simulink model "Three_phase_mf44"  (R2023b)
settings: Solver=ode45  StartTime=0.0  StopTime=0.1  RelTol=1e-3
libraries: spsDiodeLib x6, spsIdealSwitchLib x6, spsTriangleGeneratorLib x3, spsCurrentMeasurementLib x1, spsDCVoltageSourceLib x1, spsThreePhaseSeriesRLCBranchLib x1, spsVoltageMeasurementLib x1, spspowerguiLib x1
settings Model: Creator=LX  LastModifiedBy=Ngsanchong
settings DataIOCC: ReturnWorkspaceOutputs=off

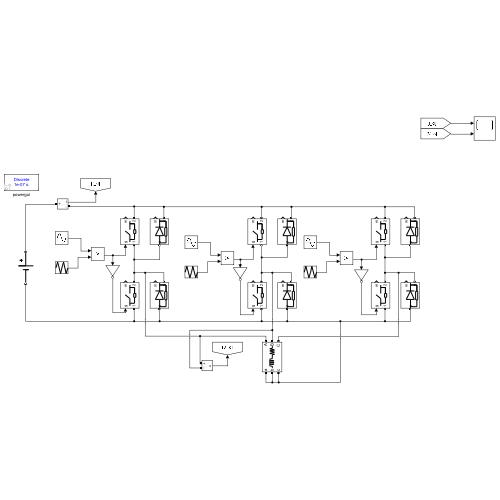
[thumbnail: Simulink's stored preview of the top-level diagram]
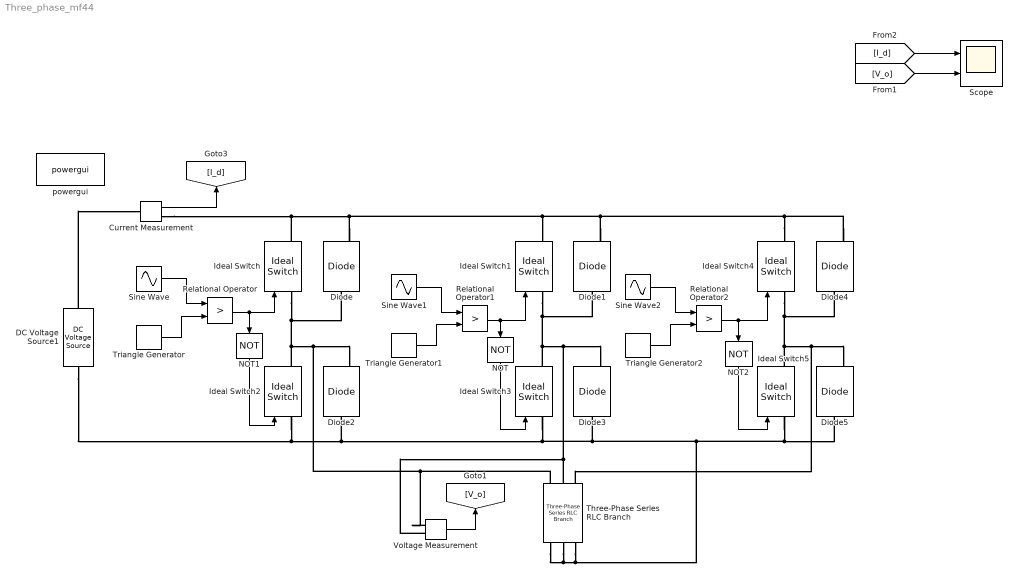
== system Three_phase_mf44 ==
  Current Measurement : spsCurrentMeasurementLib/Current Measurement  PhasorSimulation=off  OutputType=Complex  PSBequivalent=0
  DC Voltage Source1 : spsDCVoltageSourceLib/DC Voltage Source  Amplitude=540  Measurements=None
  Diode{,1..5} (6 alike) : spsDiodeLib/Diode  Ron=0.001  Lon=0  Vf=0.8  IC=0  UseSnubber=0  Rs=500  Cs=250e-9  Measurements=on
  Ideal Switch{,1..5} (6 alike) : spsIdealSwitchLib/Ideal Switch  Ron=1e-9  Lon=0  IC=0  Rs=1e5  Cs=inf  Measurements=on
  NOT : Logic  Operator=NOT  IconShape=distinctive  AllPortsSameDT=off  OutDataTypeStr=boolean
  NOT1 : Logic  Operator=NOT  IconShape=distinctive  AllPortsSameDT=off  OutDataTypeStr=boolean
  NOT2 : Logic  Operator=NOT  IconShape=distinctive  AllPortsSameDT=off  OutDataTypeStr=boolean
  Relational Operator : RelationalOperator  Operator=>  OutDataTypeStr=boolean  RndMeth=Simplest  InputSameDT=off
  Relational Operator1 : RelationalOperator  Operator=>  OutDataTypeStr=boolean  RndMeth=Simplest  InputSameDT=off
  Relational Operator2 : RelationalOperator  Operator=>  OutDataTypeStr=boolean  RndMeth=Simplest  InputSameDT=off
  Scope : Scope  NumInputPorts=2
  Sine Wave : Sin  Amplitude=1.2  Frequency=2*pi*50  SampleTime=0
  Sine Wave1 : Sin  Amplitude=1.2  Frequency=2*pi*50  Phase=-2*pi/3  SampleTime=0
  Sine Wave2 : Sin  Amplitude=1.2  Frequency=2*pi*50  Phase=2*pi/3  SampleTime=0
  Three-Phase Series RLC Branch : spsThreePhaseSeriesRLCBranchLib/Three-Phase Series RLC Branch  LConnTagsString=A|B|C  RConnTagsString=A|B|C  BranchType=RL  Resistance=5  Inductance=5e-3  Capacitance=1e-6  Measurements=None
  Triangle Generator : spsTriangleGeneratorLib/Triangle Generator  Freq=2200  Phase=90  Ts=0
  Triangle Generator1 : spsTriangleGeneratorLib/Triangle Generator  Freq=2200  Phase=90  Ts=0
  Triangle Generator2 : spsTriangleGeneratorLib/Triangle Generator  Freq=2200  Phase=90  Ts=0
  Voltage Measurement : spsVoltageMeasurementLib/Voltage Measurement  PhasorSimulation=off  OutputType=Complex  PSBequivalent=0
  powergui : spspowerguiLib/powergui  Priority=1  SimulationMode=Discrete  SampleTime=1e-7  frequency=60  Iterations=50  frequencyindice=0  Pbase=100e6  ErrMax=1e-4  UnitsV=kV  UnitsW=MW  buscounter=0  FunctionMessages=off  echomessages=off  EnableUseOfTLC=off  CurrentSourceSwitches=off  DisableSnubberDevices=off  DisableRonSwitches=off  DisableVfSwitches=off  DisplayEquations=off  AutomaticDiscreteSolvers=off  SolverType=Tustin/Backward Euler (TBE)  Interpol=off  ExternalGateDelay=off  methode=off  Ts=100  x0status=blocks  SPID=on  SwTol=0  HookPort=off  NonlinearTolerance=1e-4  nMaxIteration=100  ContinueOnMaxIteration=off  RestoreLinks=warning  ResistiveCurrentMeasurement=off  Frange=[0:2:500]  Ylog=off  Xlog=on  ShowGrid=off  save=off  variable=ZData  structure=0  ZoomFFT=off  StartTime=0.0  cycles=1  DisplayStyle=1  fundamental=60  FreqAxis=off  MaxFrequency=1000  frequencyindicesteady=1  RmsSteady=1  display=off
  wires:
  Sine Wave/1 -> Relational Operator/1
  Triangle Generator/1 -> Relational Operator/2
  Relational Operator/1 -> NOT1/1, Ideal Switch/1
  Current Measurement/1 -> [I_d]
  Voltage Measurement/1 -> [V_o]
  Triangle Generator1/1 -> Relational Operator1/2
  Sine Wave1/1 -> Relational Operator1/1
  Relational Operator1/1 -> NOT/1, Ideal Switch1/1
  NOT/1 -> Ideal Switch3/1
  NOT1/1 -> Ideal Switch2/1
  Triangle Generator2/1 -> Relational Operator2/2
  Sine Wave2/1 -> Relational Operator2/1
  NOT2/1 -> Ideal Switch5/1
  Relational Operator2/1 -> Ideal Switch4/1, NOT2/1
  [I_d] -> Scope/1
  [V_o] -> Scope/2
  connections:
  Ideal Switch4/RConn1 -- Ideal Switch/RConn1 -- Current Measurement/RConn1 -- Diode/RConn1 -- Ideal Switch1/RConn1 -- Diode1/RConn1 -- Diode4/RConn1
  Ideal Switch2/RConn1 -- Voltage Measurement/LConn1 -- Three-Phase Series RLC Branch/LConn1 -- Diode2/RConn1 -- Ideal Switch/LConn1 -- Diode/LConn1
  Ideal Switch3/RConn1 -- Ideal Switch1/LConn1 -- Diode1/LConn1 -- Three-Phase Series RLC Branch/LConn2 -- Voltage Measurement/LConn2 -- Diode3/RConn1
  Ideal Switch5/LConn1 -- Three-Phase Series RLC Branch/RConn1 -- Three-Phase Series RLC Branch/RConn2 -- Three-Phase Series RLC Branch/RConn3 -- Ideal Switch2/LConn1 -- DC Voltage Source1/LConn1 -- Diode2/LConn1 -- Ideal Switch3/LConn1 -- Diode3/LConn1 -- Diode5/LConn1
  DC Voltage Source1/RConn1 -- Current Measurement/LConn1
  Diode4/LConn1 -- Ideal Switch5/RConn1 -- Three-Phase Series RLC Branch/LConn3 -- Diode5/RConn1 -- Ideal Switch4/LConn1
